simulink subsystem "anode_subsystem_model"  (R2023a)
settings: Solver=VariableStepAuto  StartTime=0.0  StopTime=10.0  RelTol=1e-3
values from neighbouring files (symbols this model uses):
  anode_tube_D = 0.01    [anode_subsystem_parameters.m]
  N2_T = [-56.55 -50 -40 -30 -20 -10 -5 -4 -3 -2 -1 0 1 2 3 4 5 10 20 30          40 50 60 70 80 90 100 110 120 130 140 150 160 170 180 190 200 210          220 230 240 250 260 270 280 290 300 310 320 330 340 350]    [anode_subsystem_parameters.m]
libraries: fl_lib x49, nesl_utility x31, SimscapeFluids_lib x4
(part 2 of 2)

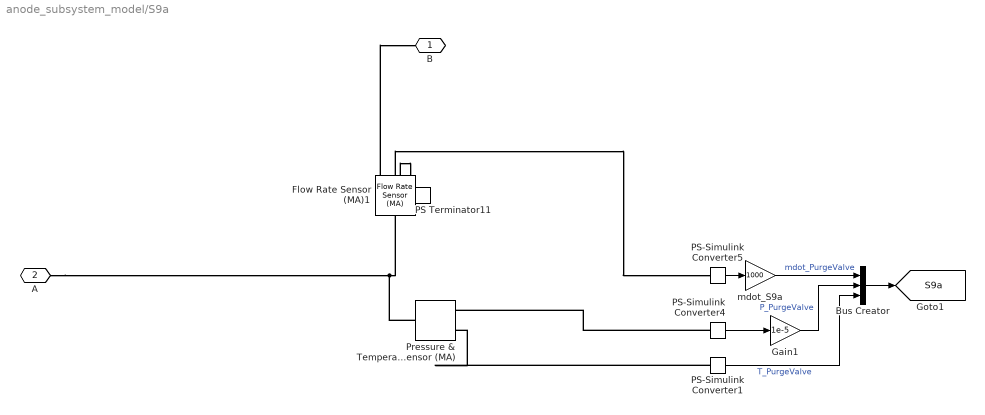
== system anode_subsystem_model/S9a ==
  Bus Creator : BusCreator  Inputs=3
  Flow Rate Sensor (MA)1 : fl_lib/Moist Air/Sensors/Flow Rate Sensor (MA)  mass_flow_measure=true  volumetric_flow_measure=false  volumetric_flow_conditions=foundation.enum.volumetric_flow_conditions.actual  p_std=0.101325 MPa  T_std=20 degC  RH_std=0.65  energy_flow_measure=true  vapor_flow_measure=false  gas_flow_measure=false
      settings: InternalSimscapePortConfiguration="{\"Bottom\":[{\"id\":\"PHI\",\"label\":\"φ\",\"type\":\"output\"}],\"Left\":[{\"id\":\"A\",\"label\":\"A\",\"type\":\"foundation.moist_air.moist_air\"}],\"Right\":[{\"id\":\"B\",\"label\":\"B\",\"type\":\"foundation.moist_air.moist_air\"},{\"id\":\"M\",\"label\":\"M\",\"type\":\"output\"}],\"Top\":[]}"
  Gain1 : Gain  Gain=1e-5
  PS Terminator11 : fl_lib/Physical Signals/Sinks/PS Terminator
  PS-Simulink Converter1 : nesl_utility/PS-Simulink Converter  PhysicalDomain=network_engine_domain  SubClassName=ps_output  LeftPortType=input  RightPortType=output  PseudoPeriodic=off  Frequencies=[]  VectorFormat=inherit  Unit=inherit  AffineConversion=off
  PS-Simulink Converter4 : nesl_utility/PS-Simulink Converter  PhysicalDomain=network_engine_domain  SubClassName=ps_output  LeftPortType=input  RightPortType=output  PseudoPeriodic=off  Frequencies=[]  VectorFormat=inherit  Unit=inherit  AffineConversion=off
  PS-Simulink Converter5 : nesl_utility/PS-Simulink Converter  PhysicalDomain=network_engine_domain  SubClassName=ps_output  LeftPortType=input  RightPortType=output  PseudoPeriodic=off  Frequencies=[]  VectorFormat=inherit  Unit=inherit  AffineConversion=off
  Pressure & Temperature Sensor (MA) : fl_lib/Moist Air/Sensors/Pressure & Temperature Sensor (MA)  reference=foundation.enum.MeasurementReference.absolute  pressure=true  pressure_spec=foundation.enum.PressureMeasementSpec.Absolute  temperature=true
      settings: InternalSimscapePortConfiguration="{\"Bottom\":[{\"id\":\"T\",\"label\":\"T\",\"type\":\"output\"}],\"Left\":[{\"id\":\"A\",\"label\":\"A\",\"type\":\"foundation.moist_air.moist_air\"}],\"Right\":[{\"id\":\"Pa\",\"label\":\"Pa\",\"type\":\"output\"}],\"Top\":[]}"
  mdot_S9a : Gain  Gain=1000
  B : PMIOPort  Side=Right
  A : PMIOPort  Port=2  Side=Left
  tag scope: S9a=global
  wires:
  Gain1/1 -> Bus Creator/2  "P_PurgeValve"
  PS-Simulink Converter1/1 -> Bus Creator/3  "T_PurgeValve"
  mdot_S9a/1 -> Bus Creator/1  "mdot_PurgeValve"
  PS-Simulink Converter5/1 -> mdot_S9a/1
  PS-Simulink Converter4/1 -> Gain1/1
  Bus Creator/1 -> [S9a]
  connections:
  A/RConn1 -- Pressure & Temperature Sensor (MA)/LConn1 -- Flow Rate Sensor (MA)1/LConn1
  Flow Rate Sensor (MA)1/RConn1 -- B/RConn1
  PS Terminator11/LConn1 -- Flow Rate Sensor (MA)1/RConn3
  Flow Rate Sensor (MA)1/RConn2 -- PS-Simulink Converter5/LConn1
  PS-Simulink Converter1/LConn1 -- Pressure & Temperature Sensor (MA)/RConn2
  PS-Simulink Converter4/LConn1 -- Pressure & Temperature Sensor (MA)/RConn1
